simulink model "DiscreteDerivative_TestGen4"  (R2017b)
settings: Solver=FixedStepDiscrete  StartTime=0.0  StopTime=10.0  RelTol=1e-3
undefined symbols (not defined in the file): Block_TestLib, enable_trigger
libraries: simulink x1
settings Model: Creator=hbourbou  LastModifiedBy=hbourbou
settings DebuggingCC: ParameterOverflowMsg=none

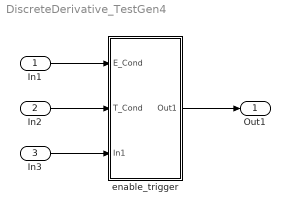
== system DiscreteDerivative_TestGen4 ==
  In1 : Inport
  In2 : Inport  Port=2
  In3 : Inport  Port=3
  enable_trigger : Subsystem  AncestorBlock=Block_TestLib/enable_trigger
  Out1 : Outport
  wires:
  In1/1 -> enable_trigger/1(E_Cond)
  In2/1 -> enable_trigger/2(T_Cond)
  In3/1 -> enable_trigger/3(In1)
  enable_trigger/1(Out1) -> Out1/1

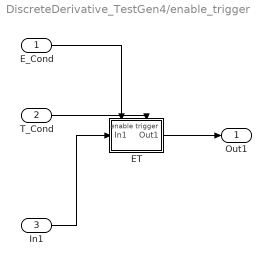
== system DiscreteDerivative_TestGen4/enable_trigger ==
  E_Cond : Inport  OutDataTypeStr=boolean
  T_Cond : Inport  Port=2  OutDataTypeStr=boolean
  In1 : Inport  Port=3
  ET : Subsystem  TreatAsAtomicUnit=on
  Out1 : Outport
  wires:
  T_Cond/1 -> ET/Trigger
  E_Cond/1 -> ET/Enable
  In1/1 -> ET/1(In1)
  ET/1(Out1) -> Out1/1

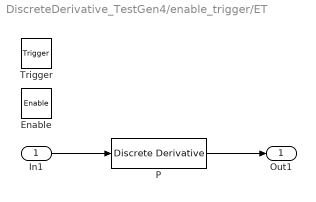
== system DiscreteDerivative_TestGen4/enable_trigger/ET ==
  In1 : Inport
  Enable : EnablePort
  Trigger : TriggerPort  VariantControl=Variant
  P : simulink/Discrete/Discrete Derivative  gainval=2.0  ICPrevScaledInput=0.0  OutMin=[]  OutMax=[]  OutDataTypeStr=uint16  OutputDataTypeScalingMode=uint16  OutDataType=fixdt(1, 16)  OutScaling=2^-10  RndMeth=Nearest  DoSatur=off
      settings: LockScale=on
  Out1 : Outport
  wires:
  In1/1 -> P/1
  P/1 -> Out1/1
